simulink model "lab2"  (R2015b)
settings: Solver=VariableStepAuto  StartTime=0.0  StopTime=1600  RelTol=1e-3
libraries: commblksprivate x1, rfmathmodels1 x1, commsynccomp2 x1, dspsigops x1
settings Model: Creator=dimple  LastModifiedBy=dimple

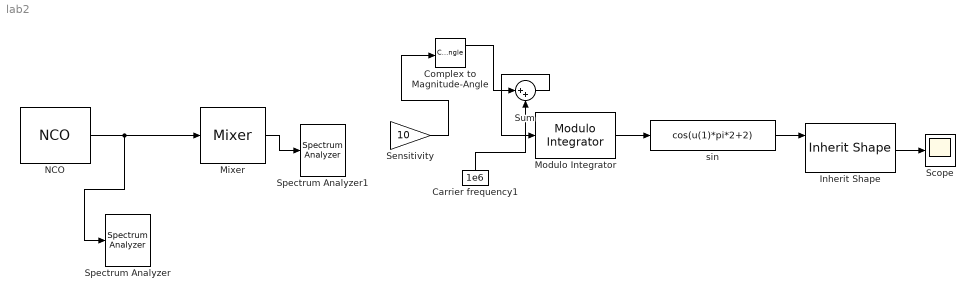
== system lab2 ==
  Carrier frequency1 : Constant  Value=1e6
  Complex to Magnitude-Angle : ComplexToMagnitudeAngle
  Inherit Shape : commblksprivate/Inherit Shape
  Mixer : rfmathmodels1/Mixer  gain=0  PhNs=-110  Fo=1e6  seed=2137  loss=0
  Modulo Integrator : commsynccomp2/Continuous-Time VCO/Modulo  Integrator  SystemSampleTime=-1
  NCO : dspsigops/NCO  AccIncSrc=Specify via dialog  AccInc=100  PhaseOffsetSrc=Specify via dialog  PhaseOffset=0  AccumWL=16  HasDither=on  DitherWL=4  PNgeneratorLength=19  HasPhaseQuantizer=on  TableDepth=12  HasOutputPhaseError=off  Formula=Complex exponential  DataType=double  OutputWL=16  OutputFL=14  CompMethod=Table lookup (no interpolation)  SampleTime=1  SamplesPerFrame=1  OutputFrames=off
  Scope : Scope
  Sensitivity : Gain  Gain=10  SaturateOnIntegerOverflow=on  OutDataTypeStr=Inherit: Same as input  ParamDataTypeStr=Inherit: Same as input
  Spectrum Analyzer : SpectrumAnalyzer
  Spectrum Analyzer1 : SpectrumAnalyzer
  Sum : Sum  Inputs=|++  SaturateOnIntegerOverflow=on  InputSameDT=on  OutDataTypeStr=Inherit: Same as first input
  sin : Fcn  Expr=cos(u(1)*pi*2+2)
  wires:
  Inherit Shape/1 -> Scope/1
  sin/1 -> Inherit Shape/1
  Sensitivity/1 -> Complex to Magnitude-Angle/1
  Carrier frequency1/1 -> Sum/2
  Modulo Integrator/1 -> sin/1
  Sum/1 -> Modulo Integrator/1
  Complex to Magnitude-Angle/1 -> Sum/1
  NCO/1 -> Spectrum Analyzer/1, Mixer/1
  Mixer/1 -> Spectrum Analyzer1/1
